simulink model "escontrol_harness"  (R2024a)
settings: Solver=VariableStepAuto  StartTime=0.0  StopTime=Tsim  FixedStep=Ts  RelTol=1e-3
undefined symbols (not defined in the file): a, a_2, b, b_2, enable_hpf, enable_hpf_2, enable_lpf, enable_lpf_2, k, k_2, phi1, phi1_2, phi2, phi2_2, theta0, theta0_2, theta_max, theta_max_2, theta_min, theta_min_2, w, w_2, w_hpf, w_hpf_2, w_lpf, w_lpf_2
settings Model: DataDictionary=escontrol.sldd  Creator=tn212  LastModifiedBy=tn212

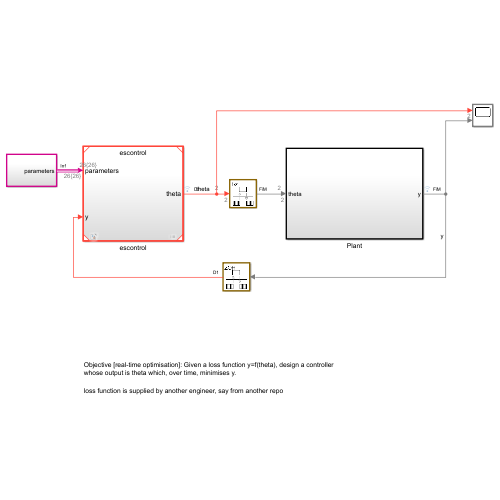
[thumbnail: Simulink's stored preview of the top-level diagram]
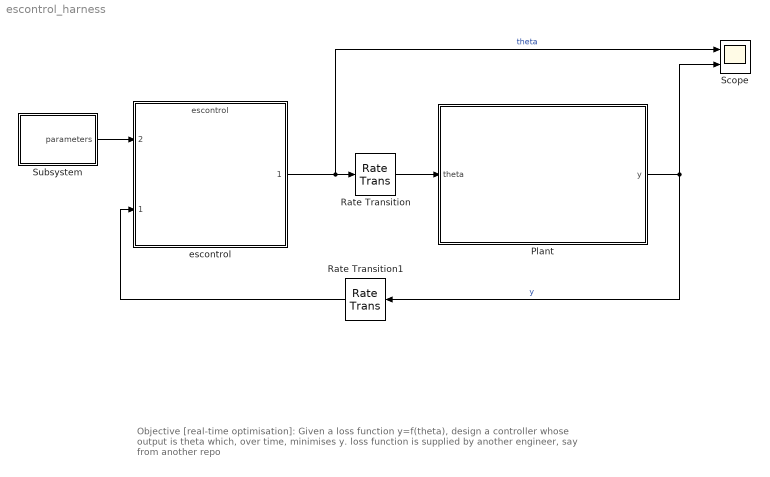
== system escontrol_harness ==
  note: Objective [real-time optimisation]: Given a loss function y=f(theta), design a controller whose output is theta which, over time, minimises y.
      |
      | loss function is supplied by another engineer, say from another repo
  Plant : Subsystem
  Rate Transition : RateTransition
  Rate Transition1 : RateTransition
  Scope : Scope  NumInputPorts=2
  Subsystem : Subsystem
  escontrol : ModelReference  ModelNameDialog=escontrol.slx  SimulationMode=Normal  ModelReferenceVersion=1.45
      settings: PortSchema="{\"entries\":[{\"content\":{\"sides\":[{\"content\":{\"connectorIds\":[\"In2\",\"In1\"]},\"type\":\"ConnectorPlacement.EquallySpacedRectSide\",\"uuid\":\"cab1f9e3-096f-40fe-9f96-b4db1ab492ca\"},{\"content\":{\"connectorIds\":[\"Out1\"],\"side\":\"RIGHT\"},\"type\":\"ConnectorPlacement.EquallySpacedRectSide\",\"uuid\":\"bf6e8ef4-d75c-497f-9a18-022bba17c823\"},{\"content\":{\"side\":\"TOP\"},\"type\":\"ConnectorPlacement.EquallySpacedRectSide\",\"uuid\":\"08acc564-e75f-4abc-b897-7c841904c396\"}]},\"type\":\"ConnectorPlacement.EquallySpacedConnector\",\"uuid\":\"37cf7a3b-eb4f-4202-acd9-6a5fb53d4501\"}],\"packageUris\":[\"http://schema.mathworks.com/mf0/Connector/R2020b\"],\"version\":\"1.0\"}"
  wires:
  Plant/1(y) -> Scope/2, Rate Transition1/1  "y"
  escontrol/1 -> Scope/1, Rate Transition/1  "theta"
  Rate Transition/1 -> Plant/1(theta)
  Subsystem/1(parameters) -> escontrol/2
  Rate Transition1/1 -> escontrol/1

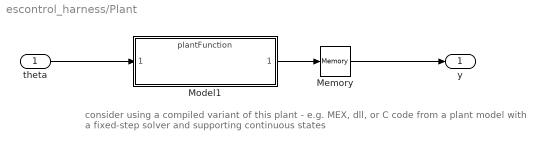
== system escontrol_harness/Plant ==
  note: consider using a compiled variant of this plant - e.g. MEX, dll, or C code from a plant model with a fixed-step solver and supporting continuous states
  theta : Inport
  Memory : Memory
  Model1 : ModelReference  ModelNameDialog=plantFunction.slx  SimulationMode=Normal  ModelReferenceVersion=1.20
  y : Outport
  wires:
  theta/1 -> Model1/1
  Model1/1 -> Memory/1
  Memory/1 -> y/1

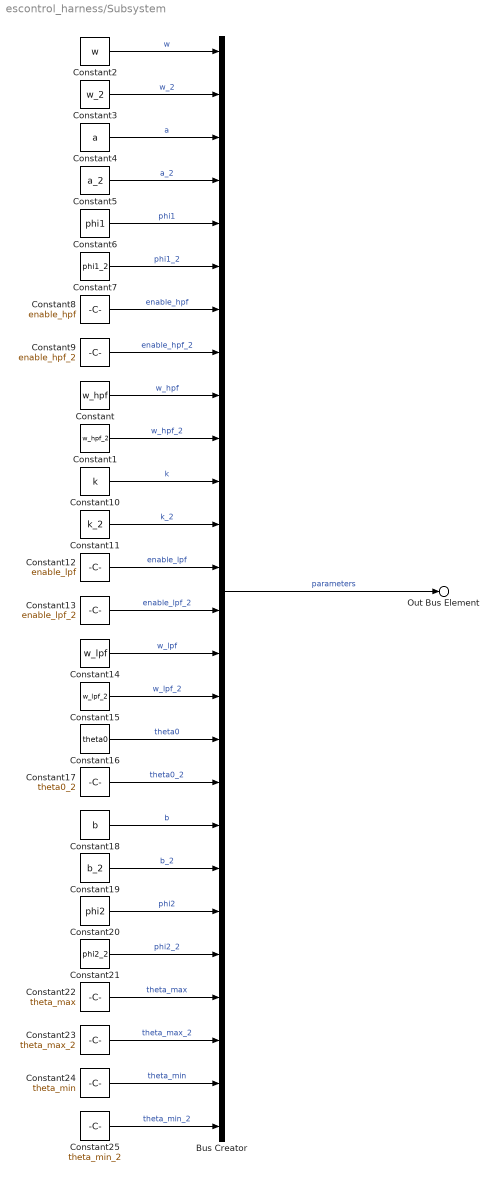
== system escontrol_harness/Subsystem ==
  Bus Creator : BusCreator  Inputs=26
  Constant : Constant  Value=w_hpf
  Constant1 : Constant  Value=w_hpf_2
  Constant10 : Constant  Value=k
  Constant11 : Constant  Value=k_2
  Constant12 : Constant  Value=enable_lpf
  Constant13 : Constant  Value=enable_lpf_2
  Constant14 : Constant  Value=w_lpf
  Constant15 : Constant  Value=w_lpf_2
  Constant16 : Constant  Value=theta0
  Constant17 : Constant  Value=theta0_2
  Constant18 : Constant  Value=b
  Constant19 : Constant  Value=b_2
  Constant2 : Constant  Value=w
  Constant20 : Constant  Value=phi2
  Constant21 : Constant  Value=phi2_2
  Constant22 : Constant  Value=theta_max
  Constant23 : Constant  Value=theta_max_2
  Constant24 : Constant  Value=theta_min
  Constant25 : Constant  Value=theta_min_2
  Constant3 : Constant  Value=w_2
  Constant4 : Constant  Value=a
  Constant5 : Constant  Value=a_2
  Constant6 : Constant  Value=phi1
  Constant7 : Constant  Value=phi1_2
  Constant8 : Constant  Value=enable_hpf
  Constant9 : Constant  Value=enable_hpf_2
  Out Bus Element : Outport  PortName=parameters
  wires:
  Constant/1 -> Bus Creator/9  "w_hpf"
  Constant1/1 -> Bus Creator/10  "w_hpf_2"
  Bus Creator/1 -> Out Bus Element/1  "parameters"
  Constant2/1 -> Bus Creator/1  "w"
  Constant3/1 -> Bus Creator/2  "w_2"
  Constant4/1 -> Bus Creator/3  "a"
  Constant5/1 -> Bus Creator/4  "a_2"
  Constant6/1 -> Bus Creator/5  "phi1"
  Constant7/1 -> Bus Creator/6  "phi1_2"
  Constant8/1 -> Bus Creator/7  "enable_hpf"
  Constant9/1 -> Bus Creator/8  "enable_hpf_2"
  Constant10/1 -> Bus Creator/11  "k"
  Constant11/1 -> Bus Creator/12  "k_2"
  Constant13/1 -> Bus Creator/14  "enable_lpf_2"
  Constant12/1 -> Bus Creator/13  "enable_lpf"
  Constant15/1 -> Bus Creator/16  "w_lpf_2"
  Constant14/1 -> Bus Creator/15  "w_lpf"
  Constant16/1 -> Bus Creator/17  "theta0"
  Constant17/1 -> Bus Creator/18  "theta0_2"
  Constant19/1 -> Bus Creator/20  "b_2"
  Constant18/1 -> Bus Creator/19  "b"
  Constant21/1 -> Bus Creator/22  "phi2_2"
  Constant20/1 -> Bus Creator/21  "phi2"
  Constant22/1 -> Bus Creator/23  "theta_max"
  Constant23/1 -> Bus Creator/24  "theta_max_2"
  Constant25/1 -> Bus Creator/26  "theta_min_2"
  Constant24/1 -> Bus Creator/25  "theta_min"
